simulink model "state_variables"  (R2024b)
settings: Solver=FixedStepDiscrete  StartTime=0.0  StopTime=10.0  FixedStep=Ts  RelTol=1e-3
undefined symbols (not defined in the file or in its folder): DiscIntNeverNeededParam
settings Model: Creator=marti  LastModifiedBy=marti

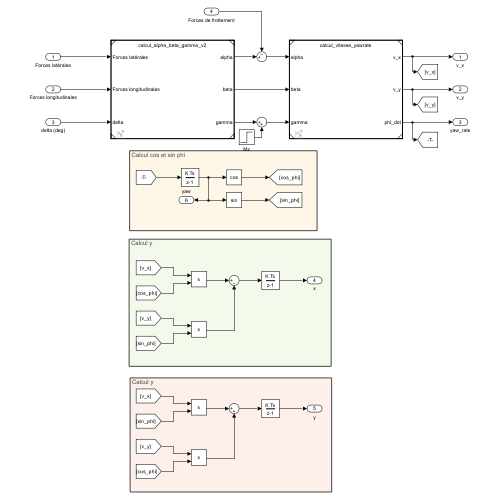
[thumbnail: Simulink's stored preview of the top-level diagram]
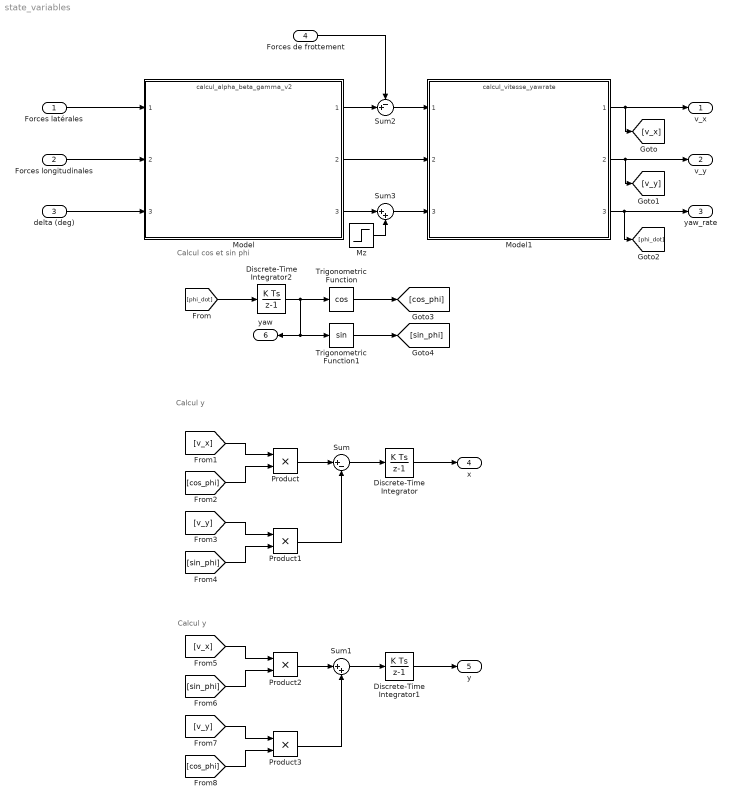
== system state_variables ==
  note: Calcul y
  note: Calcul y
  note: Calcul cos et sin phi
  Forces latérales : Inport
  Forces longitudinales : Inport  Port=2
  delta (deg) : Inport  Port=3
  Forces de frottement : Inport  Port=4
  Discrete-Time Integrator : DiscreteIntegrator  SampleTime=-1  ICPrevOutput=DiscIntNeverNeededParam  ICPrevScaledInput=DiscIntNeverNeededParam
  Discrete-Time Integrator1 : DiscreteIntegrator  SampleTime=-1  ICPrevOutput=DiscIntNeverNeededParam  ICPrevScaledInput=DiscIntNeverNeededParam
  Discrete-Time Integrator2 : DiscreteIntegrator  SampleTime=-1  ICPrevOutput=DiscIntNeverNeededParam  ICPrevScaledInput=DiscIntNeverNeededParam
  Model : ModelReference  ModelNameDialog=calcul_alpha_beta_gamma_v2.slx  SimulationMode=Normal  ModelReferenceVersion=1.6
  Model1 : ModelReference  ModelNameDialog=calcul_vitesse_yawrate.slx  SimulationMode=Normal  ModelReferenceVersion=1.3
  Mz : Step  Time=3  After=0  SampleTime=0
  Product{,1..3} (4 alike) : Product
  Sum : Sum  Inputs=|+-
  Sum1 : Sum  Inputs=|++
  Sum2 : Sum  Inputs=-+|
  Sum3 : Sum  Inputs=|++
  Trigonometric Function : Trigonometry  Operator=cos
  Trigonometric Function1 : Trigonometry
  v_x : Outport
  v_y : Outport  Port=2
  yaw_rate : Outport  Port=3
  x : Outport  Port=4
  y : Outport  Port=5
  yaw : Outport  Port=6
  wires:
  Model/2 -> Model1/2
  Forces latérales/1 -> Model/1
  delta (deg)/1 -> Model/3
  Forces longitudinales/1 -> Model/2
  Model1/1 -> [v_x], v_x/1
  Model1/2 -> [v_y], v_y/1
  Model1/3 -> [phi_dot], yaw_rate/1
  [phi_dot] -> Discrete-Time Integrator2/1
  Discrete-Time Integrator2/1 -> yaw/1, Trigonometric Function1/1, Trigonometric Function/1
  Trigonometric Function/1 -> [cos_phi]
  Trigonometric Function1/1 -> [sin_phi]
  [v_x] -> Product/1
  [cos_phi] -> Product/2
  [sin_phi] -> Product1/2
  [v_y] -> Product1/1
  Product/1 -> Sum/1
  Product1/1 -> Sum/2
  Sum/1 -> Discrete-Time Integrator/1
  [v_y] -> Product3/1
  Product2/1 -> Sum1/1
  [cos_phi] -> Product3/2
  [v_x] -> Product2/1
  Discrete-Time Integrator1/1 -> y/1
  Product3/1 -> Sum1/2
  Sum1/1 -> Discrete-Time Integrator1/1
  [sin_phi] -> Product2/2
  Model/1 -> Sum2/2
  Sum2/1 -> Model1/1
  Forces de frottement/1 -> Sum2/1
  Model/3 -> Sum3/1
  Sum3/1 -> Model1/3
  Mz/1 -> Sum3/2
  Discrete-Time Integrator/1 -> x/1
